simulink model "i2019_2_4_Suspension"  (R2017b)
settings: Solver=VariableStepAuto  StartTime=0.0  StopTime=50.0  RelTol=1e-3
values from neighbouring files (symbols this model uses):
  b1 = 350    [i2019_2_1_SystemModeling.m]    (also in i2019_2_2_SystemAnalysis.m; i2019_2_3_PID.m; i2019_2_4_Suspension_init.m)
  b2 = 15020    [i2019_2_1_SystemModeling.m]    (also in i2019_2_2_SystemAnalysis.m; i2019_2_3_PID.m; i2019_2_4_Suspension_init.m)
  k1 = 80000    [i2019_2_1_SystemModeling.m]    (also in i2019_2_2_SystemAnalysis.m; i2019_2_3_PID.m; i2019_2_4_Suspension_init.m)
  k2 = 500000    [i2019_2_1_SystemModeling.m]    (also in i2019_2_2_SystemAnalysis.m; i2019_2_3_PID.m; i2019_2_4_Suspension_init.m)
  m1 = 2500    [i2019_2_1_SystemModeling.m]    (also in i2019_2_2_SystemAnalysis.m; i2019_2_3_PID.m; i2019_2_4_Suspension_init.m)
  m2 = 320    [i2019_2_1_SystemModeling.m]    (also in i2019_2_2_SystemAnalysis.m; i2019_2_3_PID.m; i2019_2_4_Suspension_init.m)
settings Model: Creator=Joan  LastModifiedBy=joanvazq

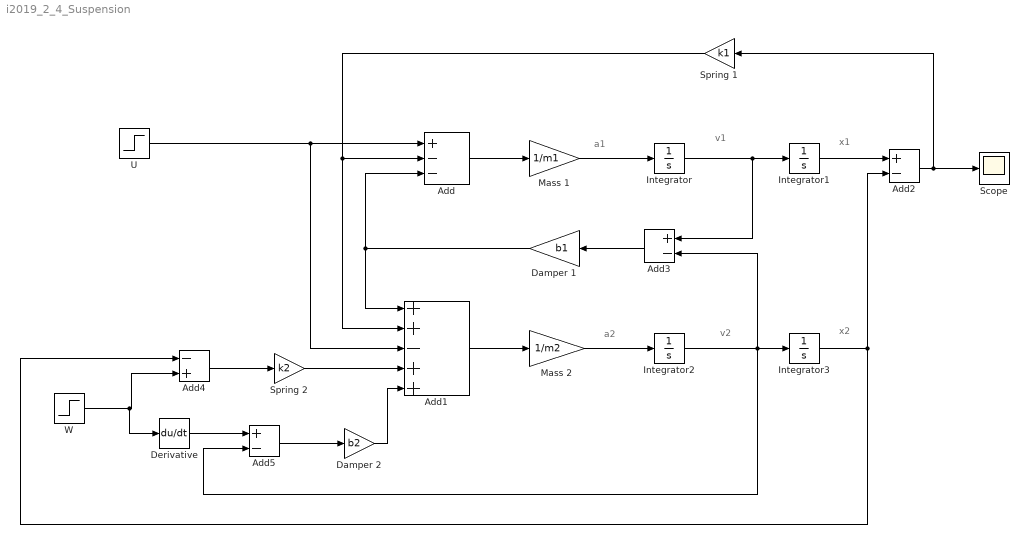
== system i2019_2_4_Suspension ==
  note: x2
  note: x1
  note: a2
  note: a1
  note: v2
  note: v1
  Add : Sum  Inputs=+--
  Add1 : Sum  Inputs=++-++
  Add2 : Sum  Inputs=+-
  Add3 : Sum  Inputs=+-
  Add4 : Sum  Inputs=-+
  Add5 : Sum  Inputs=+-
  Damper 1 : Gain  Gain=b1
  Damper 2 : Gain  Gain=b2
  Derivative : Derivative
  Integrator{,1..3} (4 alike) : Integrator
  Mass 1 : Gain  Gain=1/m1
  Mass 2 : Gain  Gain=1/m2
  Scope : Scope
  Spring 1 : Gain  Gain=k1
  Spring 2 : Gain  Gain=k2
  U : Step  Time=0  SampleTime=0
  W : Step  Time=0  After=0  SampleTime=0
  wires:
  Integrator/1 -> Add3/1, Integrator1/1
  Integrator2/1 -> Add5/2, Add3/2, Integrator3/1
  Mass 1/1 -> Integrator/1
  Mass 2/1 -> Integrator2/1
  Add/1 -> Mass 1/1
  Add1/1 -> Mass 2/1
  Integrator1/1 -> Add2/1
  Add2/1 -> Spring 1/1, Scope/1
  Spring 1/1 -> Add/2, Add1/2
  Integrator3/1 -> Add4/1, Add2/2
  Add3/1 -> Damper 1/1
  Damper 1/1 -> Add1/1, Add/3
  Spring 2/1 -> Add1/4
  Add4/1 -> Spring 2/1
  W/1 -> Derivative/1, Add4/2
  Derivative/1 -> Add5/1
  Add5/1 -> Damper 2/1
  Damper 2/1 -> Add1/5
  U/1 -> Add1/3, Add/1
